simulink model "PackDataFixed"  (R2015b)
settings: Solver=VariableStepAuto  StartTime=0.0  StopTime=10.0  RelTol=1e-3
settings Model: Creator=sk15  LastModifiedBy=sk15

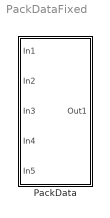
== system PackDataFixed ==
  PackData : Subsystem

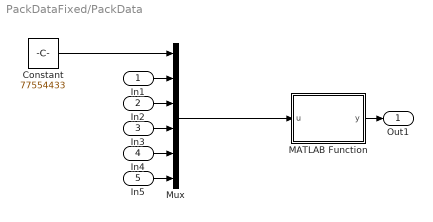
== system PackDataFixed/PackData ==
  In1 : Inport
  In2 : Inport  Port=2
  In3 : Inport  Port=3
  In4 : Inport  Port=4
  In5 : Inport  Port=5
  Constant : Constant  Value=77554433
  MATLAB Function : MATLAB Function  TreatAsAtomicUnit=on
  Mux : Mux  Inputs=6
  Out1 : Outport
  wires:
  Mux/1 -> MATLAB Function/1(u)
  Constant/1 -> Mux/1
  MATLAB Function/1(y) -> Out1/1
  In3/1 -> Mux/4
  In2/1 -> Mux/3
  In4/1 -> Mux/5
  In5/1 -> Mux/6
  In1/1 -> Mux/2

== matlab function PackDataFixed/PackData/MATLAB Function ==
  data: u input; y output
function y = fcn(u)
%#codegen

y = typecast(u,'uint8');
